simulink model "ODE_Hand_Model_v07_switching"  (Simulink 7.5)
settings: Solver=ode1  StartTime=0.0  StopTime=inf  FixedStep=0.0315/(3*12)  RelTol=1e-3
values from neighbouring files (symbols this model uses):
  K_D = 30    [Set_Parameters.m]
  K_P = 350    [Set_Parameters.m]
settings Model: Creator=nihil  LastModifiedBy=konstantinos

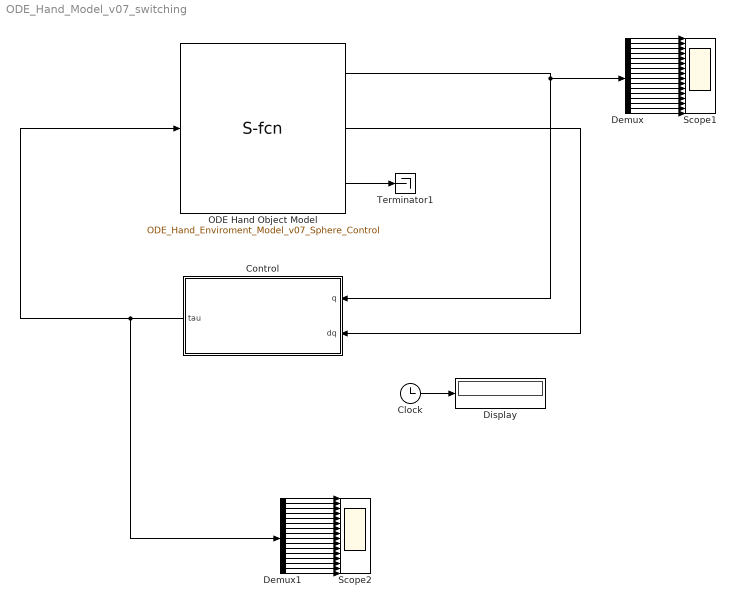
== system ODE_Hand_Model_v07_switching ==
  Clock : Clock
      settings: Decimation=10
  Control : Subsystem
  Demux : Demux  Outputs=16
  Demux1 : Demux  Outputs=16
  Display : Display
  ODE Hand Object Model : S-Function  FunctionName=ODE_Hand_Enviroment_Model_v07_Sphere_Control  EnableBusSupport=off
  Scope1 : Scope  NumInputPorts=16
      settings: YMin=-5~-5~-5~-5~-5~-5~-5~-5~-5~-5~-5~-5~-5~-5~-5~-5  YMax=5~5~5~5~5~5~5~5~5~5~5~5~5~5~5~5
  Scope2 : Scope  NumInputPorts=16
      settings: YMin=-5~-5~-5~-5~-5~-5~-5~-5~-5~-5~-5~-5~-5~-5~-5~-5  YMax=5~5~5~5~5~5~5~5~5~5~5~5~5~5~5~5
  Terminator1 : Terminator
  wires:
  Clock/1 -> Display/1
  ODE Hand Object Model/3 -> Terminator1/1
  Control/1(tau) -> ODE Hand Object Model/1, Demux1/1
  ODE Hand Object Model/1 -> Control/1(q), Demux/1
  ODE Hand Object Model/2 -> Control/2(dq)
  Demux/1 -> Scope1/1
  Demux/2 -> Scope1/2
  Demux/3 -> Scope1/3
  Demux/4 -> Scope1/4
  Demux/5 -> Scope1/5
  Demux/6 -> Scope1/6
  Demux/7 -> Scope1/7
  Demux/8 -> Scope1/8
  Demux/9 -> Scope1/9
  Demux/10 -> Scope1/10
  Demux/11 -> Scope1/11
  Demux/12 -> Scope1/12
  Demux/13 -> Scope1/13
  Demux/14 -> Scope1/14
  Demux/15 -> Scope1/15
  Demux/16 -> Scope1/16
  Demux1/1 -> Scope2/1
  Demux1/2 -> Scope2/2
  Demux1/3 -> Scope2/3
  Demux1/4 -> Scope2/4
  Demux1/5 -> Scope2/5
  Demux1/6 -> Scope2/6
  Demux1/7 -> Scope2/7
  Demux1/8 -> Scope2/8
  Demux1/9 -> Scope2/9
  Demux1/10 -> Scope2/10
  Demux1/11 -> Scope2/11
  Demux1/12 -> Scope2/12
  Demux1/13 -> Scope2/13
  Demux1/14 -> Scope2/14
  Demux1/15 -> Scope2/15
  Demux1/16 -> Scope2/16

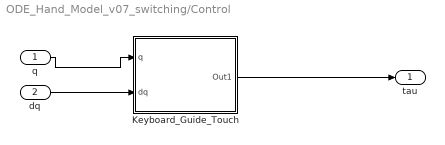
== system ODE_Hand_Model_v07_switching/Control ==
  q : Inport  OutDataType=fixdt(1, 16)  OutScaling=2^0
  dq : Inport  Port=2  OutDataType=fixdt(1, 16)  OutScaling=2^0
  Keyboard_Guide_Touch : Subsystem
  tau : Outport  OutDataType=fixdt(1, 16)  OutScaling=2^0
  wires:
  q/1 -> Keyboard_Guide_Touch/1(q)
  Keyboard_Guide_Touch/1(Out1) -> tau/1
  dq/1 -> Keyboard_Guide_Touch/2(dq)

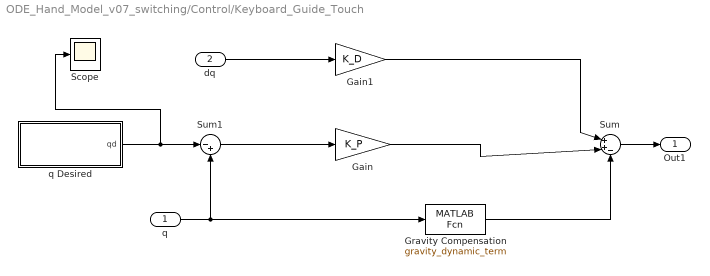
== system ODE_Hand_Model_v07_switching/Control/Keyboard_Guide_Touch ==
  q : Inport  OutDataType=fixdt(1, 16)  OutScaling=2^0
  dq : Inport  Port=2  OutDataType=fixdt(1, 16)  OutScaling=2^0
  Gain : Gain  Gain=K_P  ParameterDataType=fixdt(1, 16)  ParameterScaling=2^0  OutDataType=fixdt(1, 16)  OutScaling=2^0
  Gain1 : Gain  Gain=K_D  ParameterDataType=fixdt(1, 16)  ParameterScaling=2^0  OutDataType=fixdt(1, 16)  OutScaling=2^0
  Gravity Compensation : MATLABFcn  MATLABFcn=gravity_dynamic_term
  Scope : Scope
      settings: SaveName=ScopeData2
  Sum : Sum  Inputs=|++-  OutDataType=fixdt(1, 16)  OutScaling=2^0
  Sum1 : Sum  Inputs=|-+  OutDataType=fixdt(1, 16)  OutScaling=2^0
  q Desired : Subsystem
  Out1 : Outport  OutDataType=fixdt(1, 16)  OutScaling=2^0
  wires:
  q/1 -> Gravity Compensation/1, Sum1/2
  Sum/1 -> Out1/1
  Sum1/1 -> Gain/1
  dq/1 -> Gain1/1
  Gain1/1 -> Sum/1
  Gain/1 -> Sum/2
  q Desired/1(qd) -> Sum1/1, Scope/1
  Gravity Compensation/1 -> Sum/3

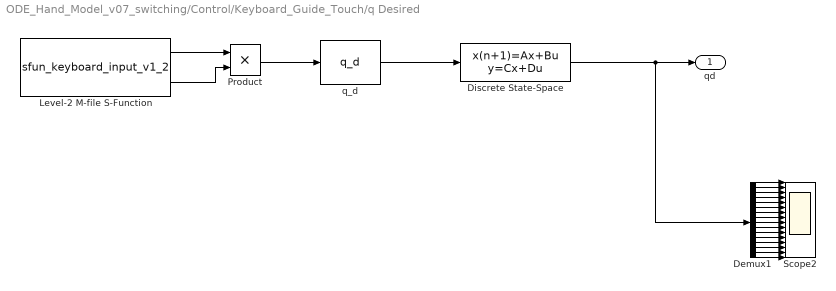
== system ODE_Hand_Model_v07_switching/Control/Keyboard_Guide_Touch/q Desired ==
  Demux1 : Demux  Outputs=16
  Discrete State-Space : DiscreteStateSpace  A=eye(16)  B=eye(16)  C=eye(16)  D=zeros(16)  X0=zeros(1,16)  SampleTime=-1
  Level-2 M-file S-Function : M-S-Function  FunctionName=sfun_keyboard_input_v1_2
  Product : Product  OutDataType=fixdt(1, 16)  OutScaling=2^0  RndMeth=Zero
  Scope2 : Scope  NumInputPorts=16
      settings: YMin=-5~-5~-5~-5~-5~-5~-5~-5~-5~-5~-5~-5~-5~-5~-5~-5  YMax=5~5~5~5~5~5~5~5~5~5~5~5~5~5~5~5  SaveName=ScopeData3
  q_d : MATLABFcn  MATLABFcn=q_d
  qd : Outport  OutDataType=fixdt(1, 16)  OutScaling=2^0
  wires:
  Level-2 M-file S-Function/2 -> Product/2
  Level-2 M-file S-Function/1 -> Product/1
  Discrete State-Space/1 -> qd/1, Demux1/1
  Product/1 -> q_d/1
  Demux1/1 -> Scope2/1
  Demux1/2 -> Scope2/2
  Demux1/3 -> Scope2/3
  Demux1/4 -> Scope2/4
  Demux1/5 -> Scope2/5
  Demux1/6 -> Scope2/6
  Demux1/7 -> Scope2/7
  Demux1/8 -> Scope2/8
  Demux1/9 -> Scope2/9
  Demux1/10 -> Scope2/10
  Demux1/11 -> Scope2/11
  Demux1/12 -> Scope2/12
  Demux1/13 -> Scope2/13
  Demux1/14 -> Scope2/14
  Demux1/15 -> Scope2/15
  Demux1/16 -> Scope2/16
  q_d/1 -> Discrete State-Space/1
